simulink model "fixedPointControllerPlant_2020b"  (R2020b)
settings: Solver=VariableStepAuto  StartTime=0.0  StopTime=10.0  RelTol=1e-3
undefined symbols (not defined in the file): data
libraries: sldrtlib x3
settings Model: Creator=fluky  LastModifiedBy=ematric
settings DebuggingCC: UnconnectedInputMsg=none  UnconnectedOutputMsg=none  UnconnectedLineMsg=none
settings ModelReferenceCC: EnableRefExpFcnMdlSchedulingChecks=off

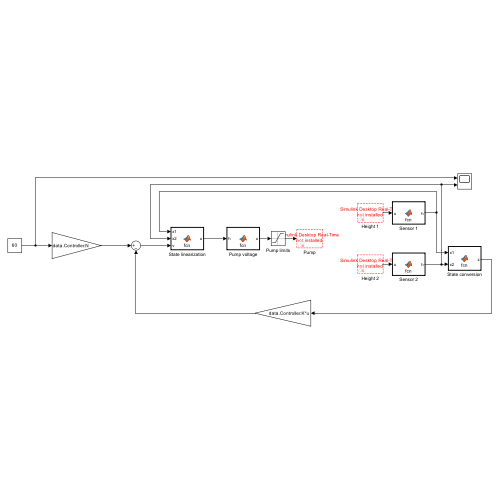
[thumbnail: Simulink's stored preview of the top-level diagram]
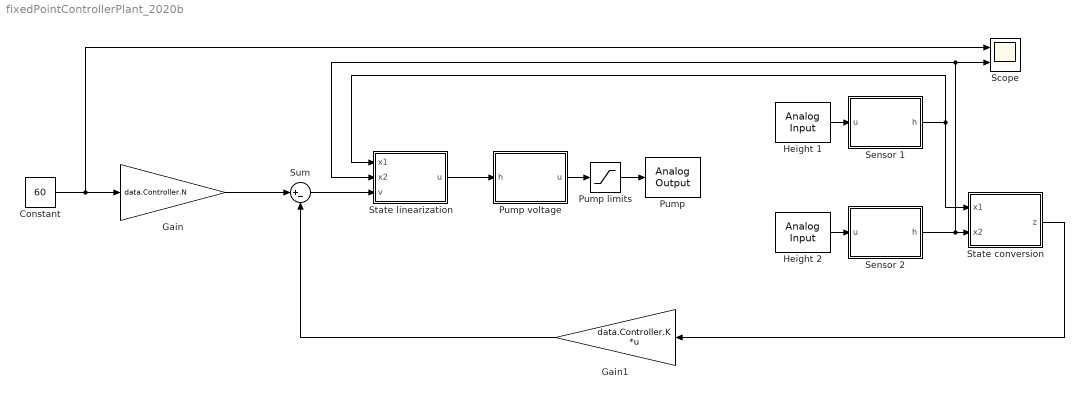
== system fixedPointControllerPlant_2020b ==
  Constant : Constant  Value=60
  Gain : Gain  Gain=data.Controller.N
  Gain1 : Gain  Gain=data.Controller.K  Multiplication=Matrix(K*u)
  Height 1 : sldrtlib/Analog Input  SampleTime=0.1  MaxMissedTicks=10  ShowMissedTicks=off  YieldWhenWaiting=off  DrvAddress=0  DrvOptions=0  Channels=1  RangeMode=1  VoltRange=1  DataType=1
  Height 2 : sldrtlib/Analog Input  SampleTime=0.1  MaxMissedTicks=10  ShowMissedTicks=off  YieldWhenWaiting=off  DrvAddress=0  DrvOptions=0  Channels=1  RangeMode=1  VoltRange=1  DataType=1
  Pump : sldrtlib/Analog Output  SampleTime=0.1  MaxMissedTicks=10  ShowMissedTicks=off  YieldWhenWaiting=off  DrvAddress=0  DrvOptions=0  Channels=1  RangeMode=1  VoltRange=1  InitialValue=[]  FinalValue=[]
  Pump limits : Saturate  UpperLimit=data.pumpMax  LowerLimit=data.pumpMin
  Pump voltage : MATLAB Function  TreatAsAtomicUnit=on
  Scope : Scope  NumInputPorts=2
  Sensor 1 : MATLAB Function  TreatAsAtomicUnit=on
  Sensor 2 : MATLAB Function  TreatAsAtomicUnit=on
  State conversion : MATLAB Function  TreatAsAtomicUnit=on
  State linearization : MATLAB Function  TreatAsAtomicUnit=on
  Sum : Sum  Inputs=|+-
  wires:
  Constant/1 -> Scope/1, Gain/1
  Gain/1 -> Sum/1
  Sum/1 -> State linearization/3(v)
  State linearization/1(u) -> Pump voltage/1(h)
  State conversion/1(z) -> Gain1/1
  Gain1/1 -> Sum/2
  Height 1/1 -> Sensor 1/1(u)
  Height 2/1 -> Sensor 2/1(u)
  Sensor 2/1(h) -> Scope/2, State linearization/2(x2), State conversion/2(x2)
  Sensor 1/1(h) -> State conversion/1(x1), State linearization/1(x1)
  Pump voltage/1(u) -> Pump limits/1
  Pump limits/1 -> Pump/1

== matlab function fixedPointControllerPlant_2020b/State conversion ==
  data: x1 input; z output; x2 input; data parameter
function z = fcn(x1, x2, data)
z = [0;0];
z(1) = x2; % is equal to y
z(2) = data.a*sqrt(x1) - data.a*sqrt(x2); % is equal to y_dot

== matlab function fixedPointControllerPlant_2020b/State linearization ==
  data: x1 input; u output; x2 input; v input; data parameter
function u = fcn(x1, x2, v, data)
u = data.roh * data.At * sqrt(x1) * (2*v/data.a + data.a*sqrt(x1/x2));

== matlab function fixedPointControllerPlant_2020b/Pump voltage ==
  data: h input; u output; data parameter
function u = fcn(h, data)
% calculation of the pump massflow
u = (h/data.rho + 2125/(210*10^6)) / (3570/(210*10^6));

== matlab function fixedPointControllerPlant_2020b/Sensor 1 ==
  data: u input; h output; data parameter
function h = fcn(u, data)
% Height = x1 * voltageSensor + x2 (x1 and x2 from polyfit)
h = data.Sensor.FitPara(1)*u + data.Sensor.FitPara(2)

== matlab function fixedPointControllerPlant_2020b/Sensor 2 ==
  data: u input; h output; data parameter
function h = fcn(u, data)
% Height = x1 * voltageSensor + x2 (x1 and x2 from polyfit)
h = data.Sensor.FitPara(1)*u + data.Sensor.FitPara(2)
